simulink library "eml_lib"  (Simulink 7.6)
settings: Solver=ode45  SolverMode=SingleTasking  StartTime=0.0  StopTime=10.0  RelTol=1e-3
settings Model: Creator=The MathWorks Inc.  ExtModeAutoUpdateStatusClock=off

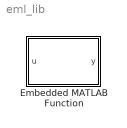
== system eml_lib ==
  Embedded MATLAB Function : Stateflow chart  TreatAsAtomicUnit=on

== matlab function Embedded MATLAB Function ==
  data: u input double; y output double
function y = fcn(u)
%#eml

y = u;
